simulink model "UARTSerialParalel"  (R2017b)
settings: Solver=VariableStepAuto  StartTime=0.0  StopTime=1  RelTol=1e-3
libraries: instrumentlib x2, simulink x1
settings Model: Creator=pipe  LastModifiedBy=pipe

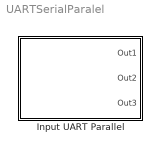
== system UARTSerialParalel ==
  Input UART Parallel : Subsystem

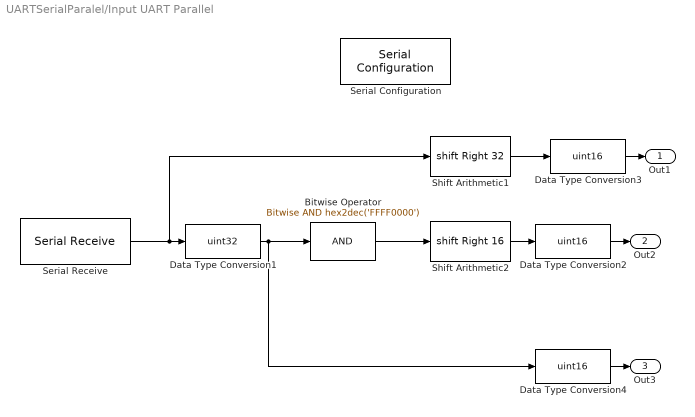
== system UARTSerialParalel/Input UART Parallel ==
  Bitwise Operator : simulink/Logic and Bit Operations/Bitwise Operator  logicop=AND  UseBitMask=on  BitMask=hex2dec('FFFF0000')  BitMaskRealWorld=Stored Integer
  Data Type Conversion1 : DataTypeConversion  OutDataTypeStr=uint32
  Data Type Conversion2 : DataTypeConversion  OutDataTypeStr=uint16
  Data Type Conversion3 : DataTypeConversion  OutDataTypeStr=uint16
  Data Type Conversion4 : DataTypeConversion  OutDataTypeStr=uint16
  Serial Configuration : instrumentlib/Serial Configuration  Priority=-200000  ComPortMenu=<Please select a port...>  ComPort=<Please select a port...>  BaudRate=9600  DataBits=8  Parity=none  StopBits=1  FlowControl=none  Timeout=10  ByteOrder=LittleEndian
  Serial Receive : instrumentlib/Serial Receive  ComPortMenu=<Please select a port...>  ComPort=<Please select a port...>  Terminator=<none>  DataSize=[1 1]  DataType=uint8  EnableBlockingMode=on  ActionDataUnavailable=Output last received value  CustomValue=0  SampleTime=0.01
  Shift Arithmetic1 : ArithShift  BitShiftNumber=32  BitShiftDirection=Right
  Shift Arithmetic2 : ArithShift  BitShiftNumber=16  BitShiftDirection=Right
  Out1 : Outport
  Out2 : Outport  Port=2
  Out3 : Outport  Port=3
  wires:
  Shift Arithmetic1/1 -> Data Type Conversion3/1
  Shift Arithmetic2/1 -> Data Type Conversion2/1
  Serial Receive/1 -> Shift Arithmetic1/1, Data Type Conversion1/1
  Bitwise Operator/1 -> Shift Arithmetic2/1
  Data Type Conversion4/1 -> Out3/1
  Data Type Conversion3/1 -> Out1/1
  Data Type Conversion2/1 -> Out2/1
  Data Type Conversion1/1 -> Data Type Conversion4/1, Bitwise Operator/1
